simulink model "test_PCI6251_20130416_3ch"  (Simulink 7.7)
settings: Solver=ode4  StartTime=0.0  StopTime=inf  RelTol=1e-3
PreLoadFcn:
  | % Here are parameters fixed
  | % during running the real-time programs.
  | %
  | winLen=256;
  | ana_hopSize=44;
  | syn_hopSize=90;
  | 
  | nFFT=1024;
  | SampRate=44100;
  | Ts=1/SampRate;
  | 
  | % % now encoded in RealSong_control
  | %cepst_nfft=2048;    % nfft size for cepstrum.
  | %
  | %up_pitch= 8000;%
  | %low_pitch=400;%
  | %
  | %quefrency = [0:cepst_nfft]'*nFFT/(SampRate*cepst_nfft); % quefrency in [sec].
  | %quefrency_index=find((1./quefrency<up_pitch & 1./quefrency > low_pitch)); % select quefrency in 400 to 8000 Hz range.
  | 
  | 
  | %frange=[400,8000];
  | %f=SampRate*((1:nFFT)-1)/nFFT;
  | %findex=find(f>=frange(1)&f<=frange(2));
  | %entropy_frange=[1000,8000];
  | %efindex=find(f>=entropy_frange(1)&f<=entropy_frange(2));
  | 
  | 
  | mingap=1;
  | minsyl =6;
values from neighbouring files (symbols this model uses):
  amp_thresh = str2double(get(handles.edit_amp_thresh,'String'))    [RealSong_control_013.m]
  efindex = find(f>=efrange(1)&f<=efrange(2))    [RealSong_control_013.m]
  findex = find(f>=pm.frange(1)&f<=pm.frange(2))    [RealSong_control_013.m]
  mainsyl = varargin{1}    [RealSong_control_013.m]
  quefrency_index = find((1./quefrency<up_pitch & 1./quefrency > low_pitch))    [RealSong_control_013.m]
  scaling_factor = presyl.template_scaling_factor    [RealSong_control_013.m]
undefined symbols (not defined in the file or in its folder): AO1_TTL_Freq, dfilt, init_stim_vector, maindetection_startcnt, maintarget_spectrum_filter, max_presyl_cancel_counter, presyl_cntmin, svmdata
libraries: simulink x13, dspsigops x4, xpcnilib x3, dsparch4 x2, dspxfrm3 x2, IntelSMIlibR2007b x1
(part 1 of 2)
settings Model: Creator=hammer  LastModifiedBy=mooney_lab  BufferReuse=off
settings OptimizationCC: BlockReduction=off  OptimizeBlockIOStorage=off  BufferReuse=off  ExpressionFolding=off  LocalBlockOutputs=off
settings DebuggingCC: UnderspecifiedInitializationDetection=Simplified
settings HardwareCC: ProdIntDivRoundTo=Zero  ProdEndianess=LittleEndian  ProdHWDeviceType=Generic->32-bit x86 compatible
settings RTWCC: SystemTargetFile=xpctarget.tlc  TemplateMakefile=xpc_default_tmf  Description=xPC Target  RTWVerbose=off  ProcessScript=xpctarget_make_rtw_hook  RTWCompilerOptimization=On
settings xpcTargetCC: TargetFcnLib=ansi_tfl_table_tmw.mat  TargetFunctionLibrary=XPC_BLAS  FunctionExecutionProfile=off  CodeExecutionProfiling=off  ERTCodeCoverageTool=None  ParMdlRefBuildCompliant=on  CombineSignalStateStructs=off  PortableWordSizes=off  xPCTaskExecutionProfile=off  xPCRL32EventNumber=5000  xPCLoadParamSetFile=off  xPCConcurrentTasks=off  xPCEnableSFAnimation=off

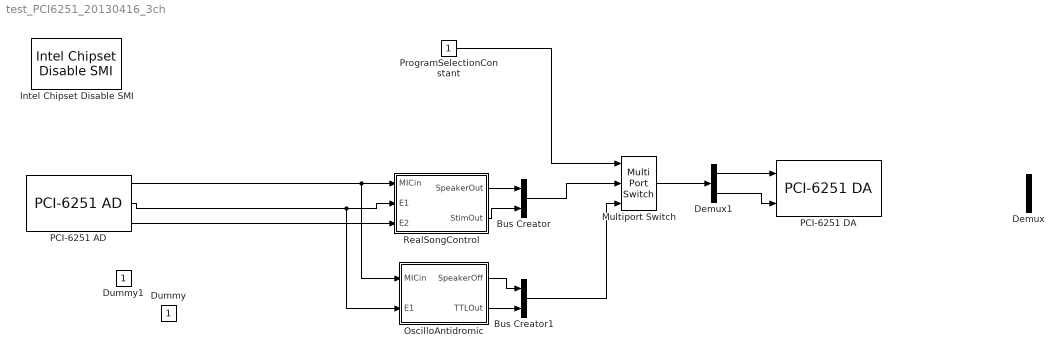
== system test_PCI6251_20130416_3ch ==
  Bus Creator : BusCreator  Inputs=2
  Bus Creator1 : BusCreator  Inputs=2
  Demux : Demux  Outputs=2
  Demux1 : Demux  Outputs=2
  Dummy : Constant  SampleTime=Ts
  Dummy1 : Constant  SampleTime=Ts
  Intel Chipset Disable SMI : IntelSMIlibR2007b/Intel Chipset Disable SMI
  Multiport Switch : MultiPortSwitch  Inputs=2  zeroidx=off
  OscilloAntidromic : Subsystem
  PCI-6251 AD : xpcnilib/A//D/M Series/PCI-6251 AD  channel=[1,2,3]  range=[10 10 10]  coupling=[0 0 0]  scantime=[4e-6, 4e-6, 4e-6]  sampletime=Ts  slot=-1
  PCI-6251 DA : xpcnilib/D//A/M Series/PCI-6251 DA  channel=[1,2]  range=[10, 10]  reset=[1, 1]  initValue=[0, 0]  sampletime=Ts  slot=-1
  ProgramSelectionConstant : Constant  SampleTime=Ts
  RealSongControl : Subsystem
  wires:
  PCI-6251 AD/1 -> RealSongControl/1(MICin), OscilloAntidromic/1(MICin)
  ProgramSelectionConstant/1 -> Multiport Switch/1
  RealSongControl/1(SpeakerOut) -> Bus Creator/1
  RealSongControl/2(StimOut) -> Bus Creator/2
  OscilloAntidromic/1(SpeakerOff) -> Bus Creator1/1
  OscilloAntidromic/2(TTLOut) -> Bus Creator1/2
  Bus Creator/1 -> Multiport Switch/2
  Bus Creator1/1 -> Multiport Switch/3
  Multiport Switch/1 -> Demux1/1
  Demux1/1 -> PCI-6251 DA/1
  Demux1/2 -> PCI-6251 DA/2
  PCI-6251 AD/2 -> RealSongControl/2(E1), OscilloAntidromic/2(E1)
  PCI-6251 AD/3 -> RealSongControl/3(E2)

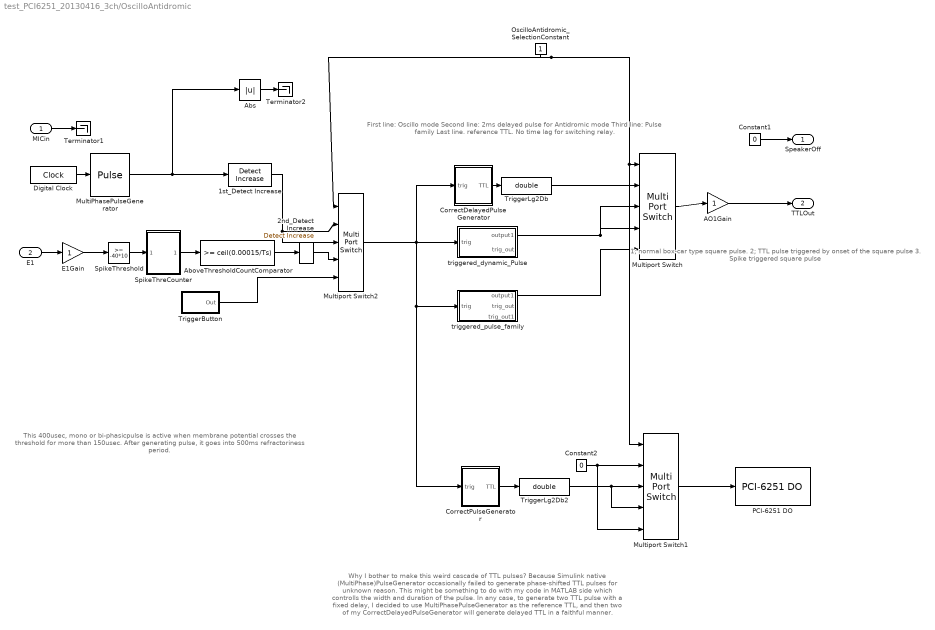
== system test_PCI6251_20130416_3ch/OscilloAntidromic ==
  note: 1; normal box-car type square pulse.
      | 2; TTL pulse triggered by onset of the square pulse
      | 3. Spike triggered square pulse
  note: First line: Oscillo mode
      | Second line: 2ms delayed pulse for Antidromic mode
      | Third line: Pulse family
      | Last line. reference TTL. No time lag for switching relay.
  note: Why I bother to make this weird cascade of TTL pulses?
      | Because Simulink native (MultiPhase)PulseGenerator occasionally failed
      | to generate phase-shifted TTL pulses for unknown reason.
      | This might be something to do with my code in MATLAB side which
      | controlls the width and duration of the pulse. In any case,
      |  to generate two TTL pulse with a fixed delay,
      | I decided to use MultiPhasePulseGenerator as the reference TTL,
      | and then two of my CorrectDelayedPulseGenerator
      | will generate delayed TTL in a faithful manner.
  note: This 400usec, mono or bi-phasicpulse is
      | active when membrane potential crosses the threshold
      | for more than 150usec. After generating pulse,
      | it goes into 500ms refractoriness period.
  MICin : Inport
  E1 : Inport  Port=2
  1st_Detect Increase : simulink/Logic and Bit Operations/Detect Increase  SystemSampleTime=-1  vinit=0.0
  2nd_Detect Increase : simulink/Logic and Bit Operations/Detect Increase  SystemSampleTime=-1  vinit=0.0
  AO1Gain : Gain
  AboveThresholdCountComparator : simulink/Logic and Bit Operations/Compare To Constant  SystemSampleTime=-1  relop=>=  const=ceil(0.00015/Ts)  LogicOutDataTypeMode=uint8
  Abs : Abs
  Constant1 : Constant  Value=0
  Constant2 : Constant  Value=0
  CorrectDelayedPulseGenerator : Subsystem  mask{maindetection_startcnt=ceil(0.002/Ts), width=ceil(0.05/Ts)}
      mask prompts: maindetection_startcnt "Delay (count)"; width "Width of TTL (count)"
  CorrectPulseGenerator : Subsystem  mask{maindetection_startcnt=0, width=ceil(0.05/Ts)}
      mask prompts: maindetection_startcnt "Delay (count)"; width "Width of TTL (count)"
  Digital Clock : DigitalClock  SampleTime=Ts
  E1Gain : Gain
  MultiPhasePulseGenerator : DiscretePulseGenerator  TimeSource=Use external signal  Period=ceil(1/AO1_TTL_Freq/Ts)  PulseWidth=ceil(0.5/AO1_TTL_Freq/Ts)  SampleTime=Ts
  Multiport Switch : MultiPortSwitch  Inputs=4  zeroidx=off
  Multiport Switch1 : MultiPortSwitch  Inputs=4  zeroidx=off
  Multiport Switch2 : MultiPortSwitch  Inputs=4  zeroidx=off
  OscilloAntidromic_SelectionConstant : Constant  SampleTime=Ts
  PCI-6251 DO : xpcnilib/Digital Output/M Series/PCI-6251 DO  channel=[1]  reset=[1]  initValue=[0]  sampletime=Ts  slot=-1
  SpikeThreCounter : Subsystem
  SpikeThreshold : simulink/Logic and Bit Operations/Compare To Constant  SystemSampleTime=-1  relop=>=  const=-40*10  LogicOutDataTypeMode=uint8
      link override Compare: Operator=<=
  Terminator1 : Terminator
  Terminator2 : Terminator
  TriggerButton : Subsystem
  TriggerLg2Db : DataTypeConversion  OutDataTypeStr=double  RndMeth=Zero
  TriggerLg2Db2 : DataTypeConversion  OutDataTypeStr=double  RndMeth=Zero
  triggered_dynamic_Pulse : Subsystem  mask{amp=1, delay=ceil(0.001/Ts), pulse_dur=ceil(0.0002/Ts), ipi=ceil(0.00021/Ts), burst_dur=ceil(0.00042/Ts), ref=ceil(0.5/Ts)}
      mask prompts: amp "Amp [V]"; delay "delay [ms]"; pulse_dur "pulse duration  [ms]"; ipi "inter_pulse_interval  [ms]"; burst_dur "total burst duration  [ms]"; ref "Ref  [ms]"
      mask init:
      | Y = make_pulse(delay,burst_dur,pulse_dur,ipi,1,44100);
      | X = 1:length(Y);
      mask Display: plot(X,Y)
  triggered_pulse_family : Subsystem  mask{delay=ceil(0.1/Ts), pulse_dur=ceil(0.1/Ts), ipi=ceil(0.4/Ts), burst_dur=ceil(1/Ts), ref=ceil(1/Ts), lowamp=-600, interval=600, highamp=600}
      mask prompts: delay "delay [ms]"; pulse_dur "pulse duration  [ms]"; ipi "inter_pulse_interval  [ms]"; burst_dur "total burst duration  [ms]"; ref "Ref  [ms]"; lowamp "Lowest current [pA]"; interval "current interval [pA]"; highamp "Highest current [pA]"
      mask init:
      | amp=[lowamp:interval:highamp]
      | if ceil(burst_dur/ipi)>length(amp)
      |     errordlg(sprintf('amp vector (%d)is shorter than required length (%d)!',...
      |         length(amp),ceil(burst_dur/ipi)));
      | end
      | 
      | Y = make_pulsefamily(delay,burst_dur,pulse_dur,ipi,amp,44100);
      | X = 1:length(Y);
      mask Display: plot(X,Y)
  SpeakerOff : Outport
  TTLOut : Outport  Port=2
  wires:
  Constant1/1 -> SpeakerOff/1
  AO1Gain/1 -> TTLOut/1
  E1/1 -> E1Gain/1
  E1Gain/1 -> SpikeThreshold/1
  MICin/1 -> Terminator1/1
  OscilloAntidromic_SelectionConstant/1 -> Multiport Switch/1, Multiport Switch1/1, Multiport Switch2/1
  Multiport Switch/1 -> AO1Gain/1
  triggered_dynamic_Pulse/1(output1) -> Multiport Switch/3, Multiport Switch/4
  Constant2/1 -> Multiport Switch1/2, Multiport Switch1/5
  Multiport Switch1/1 -> PCI-6251 DO/1
  Digital Clock/1 -> MultiPhasePulseGenerator/1
  CorrectDelayedPulseGenerator/1(TTL) -> TriggerLg2Db/1
  TriggerLg2Db/1 -> Multiport Switch/2
  TriggerLg2Db2/1 -> Multiport Switch1/4, Multiport Switch1/3
  SpikeThreshold/1 -> SpikeThreCounter/1(LogicalInput)
  SpikeThreCounter/1(count) -> AboveThresholdCountComparator/1
  Multiport Switch2/1 -> CorrectDelayedPulseGenerator/1(trig), CorrectPulseGenerator/1(trig), triggered_pulse_family/1(trig), triggered_dynamic_Pulse/1(trig)
  MultiPhasePulseGenerator/1 -> 1st_Detect Increase/1, Abs/1
  CorrectPulseGenerator/1(TTL) -> TriggerLg2Db2/1
  AboveThresholdCountComparator/1 -> 2nd_Detect Increase/1
  triggered_pulse_family/1(output1) -> Multiport Switch/5
  TriggerButton/1(Out) -> Multiport Switch2/5
  1st_Detect Increase/1 -> Multiport Switch2/3, Multiport Switch2/2
  2nd_Detect Increase/1 -> Multiport Switch2/4
  Abs/1 -> Terminator2/1

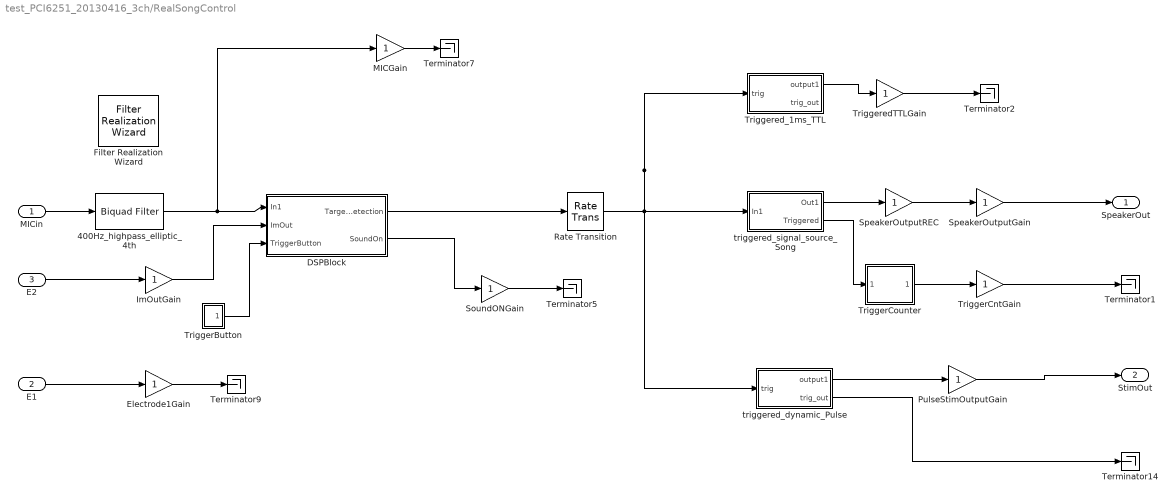
== system test_PCI6251_20130416_3ch/RealSongControl ==
  MICin : Inport
  E1 : Inport  Port=2
  E2 : Inport  Port=3
  400Hz_highpass_elliptic_4th : dsparch4/Biquad Filter  Tag=BlockMethodSubSystem  IIRFiltStruct=Direct form II  CoeffSource=Specify via dialog  BiQuadCoeffs=[1 -1.99997295416341 1 1 -1.86330921959673 0.873887398426786;1 -1.99984550773747 1 1 -1.98119934202051 0.984460391369785]  a0Flag=Warning  IC=0  ICnum=0  ICden=0  InputProcessing=Columns as channels (frame based)  denAccumFracLength=30  denProdOutputFracLength=30  secondMemoryFracLength=15  roundingMode=Floor  overflowMode=off  ScaleValues=[16.3731438660539;0.0504230422181438;1]  optimizeScaleValues=on  ScaleValueMode=Specify via input port (g)  scaleValueFracLength=14  FilterSource=Specify via dialog  dfiltObjectName=dfilt.df2tsos([1 0.3 0.4],[1 0.1 0.2])
  DSPBlock : Subsystem
  Electrode1Gain : Gain
  Filter Realization Wizard : dsparch4/Filter Realization Wizard  SystemSampleTime=-1
  ImOutGain : Gain
  MICGain : Gain
  PulseStimOutputGain : Gain
  Rate Transition : RateTransition
  SoundONGain : Gain
  SpeakerOutputGain : Gain
  SpeakerOutputREC : Gain
  Terminator{1..2,5,7,9,14} (6 alike) : Terminator
  TriggerButton : Subsystem
  TriggerCntGain : Gain
  TriggerCounter : Subsystem
  TriggeredTTLGain : Gain
  Triggered_1ms_TTL : Subsystem  mask{amp=1, delay=0.0, pulse_dur=ceil(1/1000*SampRate), ipi=ceil(1/1000*SampRate), burst_dur=ceil(1/1000*SampRate), ref=ceil(1/1000*SampRate)}
      mask prompts: amp "Amp [V]"; delay "delay [ms]"; pulse_dur "pulse duration  [ms]"; ipi "inter_pulse_interval  [ms]"; burst_dur "total burst duration  [ms]"; ref "Ref  [ms]"
      mask init:
      | Y = make_pulse(delay,burst_dur,pulse_dur,ipi,1,44100);
      | X = 1:length(Y);
      mask Display: plot(X,Y)
  triggered_dynamic_Pulse : Subsystem  mask{amp=1, delay=0, pulse_dur=ceil(0.4/1000*SampRate), ipi=ceil(1/1000*SampRate), burst_dur=ceil(4/1000*SampRate), ref=ceil(100/1000*SampRate)}
      mask prompts: amp "Amp [V]"; delay "delay [ms]"; pulse_dur "pulse duration  [ms]"; ipi "inter_pulse_interval  [ms]"; burst_dur "total burst duration  [ms]"; ref "Ref  [ms]"
      mask init:
      | Y = make_pulse(delay,burst_dur,pulse_dur,ipi,1,44100);
      | X = 1:length(Y);
      mask Display: plot(X,Y)
  triggered_signal_source_Song : Subsystem  mask{OutValues=init_stim_vector, ref=length(init_stim_vector), on_off=1}
      mask prompts: OutValues "Output Values"; on_off "ON/Off"
      mask init:
      | dim = size(OutValues);
      | if length(dim) > 2 || min(dim) ~= 1
      |   [X, Y] =  generateQuestionMarkIconData;
      | error('Parameter ''output values'' must be a vector or a scalar');
      |   else
      |   nn = length(OutValues);
      |   xx = (0:nn);
      |   yy = double([reshape(OutValues,1,nn) OutValues(end)]);
      |  X = fixpt_look1_mask_data(xx,yy,1,4);
      |  Y = fixpt_look1_mask_data(xx,yy,0,4);
      |  end
      mask Display: plot(X,Y)
  SpeakerOut : Outport
  StimOut : Outport  Port=2
  wires:
  triggered_signal_source_Song/1(Out1) -> SpeakerOutputREC/1
  triggered_signal_source_Song/2(Triggered) -> TriggerCounter/1(LogicalInput)
  TriggerCounter/1(count) -> TriggerCntGain/1
  MICGain/1 -> Terminator7/1
  SpeakerOutputGain/1 -> SpeakerOut/1
  E1/1 -> Electrode1Gain/1
  Electrode1Gain/1 -> Terminator9/1
  PulseStimOutputGain/1 -> StimOut/1
  triggered_dynamic_Pulse/1(output1) -> PulseStimOutputGain/1
  triggered_dynamic_Pulse/2(trig_out) -> Terminator14/1
  SoundONGain/1 -> Terminator5/1
  TriggerCntGain/1 -> Terminator1/1
  TriggeredTTLGain/1 -> Terminator2/1
  Triggered_1ms_TTL/1(output1) -> TriggeredTTLGain/1
  DSPBlock/2(SoundOn) -> SoundONGain/1
  400Hz_highpass_elliptic_4th/1 -> DSPBlock/1(In1), MICGain/1
  MICin/1 -> 400Hz_highpass_elliptic_4th/1
  SpeakerOutputREC/1 -> SpeakerOutputGain/1
  Rate Transition/1 -> triggered_dynamic_Pulse/1(trig), triggered_signal_source_Song/1(In1), Triggered_1ms_TTL/1(trig)
  TriggerButton/1(Out1) -> DSPBlock/3(TriggerButton)
  E2/1 -> ImOutGain/1
  ImOutGain/1 -> DSPBlock/2(ImOut)
  DSPBlock/1(TargetSyllableDetection) -> Rate Transition/1

== system test_PCI6251_20130416_3ch/OscilloAntidromic/CorrectDelayedPulseGenerator ==
  trig : Inport
  Delayed TTL generator : Stateflow chart  TreatAsAtomicUnit=on
  delay : Constant  Value=maindetection_startcnt  VectorParams1D=off
  width : Constant  Value=width  VectorParams1D=off
  TTL : Outport
  wires:
  delay/1 -> Delayed TTL generator/2(delays)
  width/1 -> Delayed TTL generator/3(width)
  trig/1 -> Delayed TTL generator/1(trig)
  Delayed TTL generator/1(out) -> TTL/1

== system test_PCI6251_20130416_3ch/OscilloAntidromic/CorrectPulseGenerator ==
  trig : Inport
  Delayed TTL generator : Stateflow chart  TreatAsAtomicUnit=on
  delay : Constant  Value=maindetection_startcnt  VectorParams1D=off
  width : Constant  Value=width  VectorParams1D=off
  TTL : Outport
  wires:
  delay/1 -> Delayed TTL generator/2(delays)
  width/1 -> Delayed TTL generator/3(width)
  trig/1 -> Delayed TTL generator/1(trig)
  Delayed TTL generator/1(out) -> TTL/1

== system test_PCI6251_20130416_3ch/OscilloAntidromic/SpikeThreCounter ==
  LogicalInput : Inport
  Counter : Subsystem  TreatAsAtomicUnit=on
  Data Type Conversion1 : DataTypeConversion  OutDataTypeStr=double  RndMeth=Zero
  count : Outport
  wires:
  Data Type Conversion1/1 -> Counter/1(In1)
  LogicalInput/1 -> Data Type Conversion1/1, Counter/Enable
  Counter/1(Out1) -> count/1

== system test_PCI6251_20130416_3ch/OscilloAntidromic/TriggerButton ==
  Detect Change : simulink/Logic and Bit Operations/Detect Change  SystemSampleTime=-1  vinit=1.0
  TrigVal : Constant  Value=1.0  OutDataTypeStr=int8
  TriggerLg2Db : DataTypeConversion  OutDataTypeStr=double  RndMeth=Zero
  Out : Outport
  wires:
  Detect Change/1 -> TriggerLg2Db/1
  TrigVal/1 -> Detect Change/1
  TriggerLg2Db/1 -> Out/1

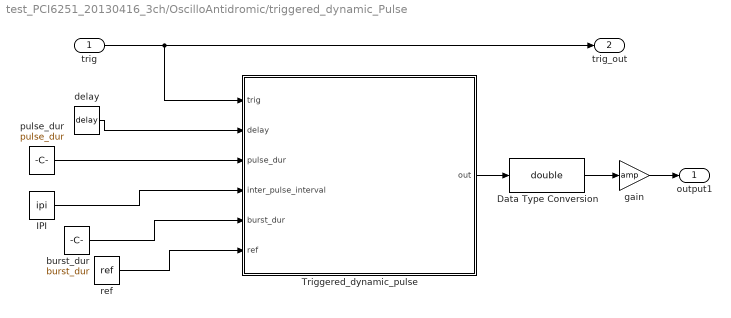
== system test_PCI6251_20130416_3ch/OscilloAntidromic/triggered_dynamic_Pulse ==
  trig : Inport
  Data Type Conversion : DataTypeConversion  OutDataTypeStr=double
  IPI : Constant  Value=ipi
  Triggered_dynamic_pulse : Stateflow chart  TreatAsAtomicUnit=on
  burst_dur : Constant  Value=burst_dur
  delay : Constant  Value=delay
  gain : Gain  Gain=amp
  pulse_dur : Constant  Value=pulse_dur
  ref : Constant  Value=ref
  output1 : Outport
  trig_out : Outport  Port=2
  wires:
  delay/1 -> Triggered_dynamic_pulse/2(delay)
  pulse_dur/1 -> Triggered_dynamic_pulse/3(pulse_dur)
  IPI/1 -> Triggered_dynamic_pulse/4(inter_pulse_interval)
  burst_dur/1 -> Triggered_dynamic_pulse/5(burst_dur)
  ref/1 -> Triggered_dynamic_pulse/6(ref)
  trig/1 -> Triggered_dynamic_pulse/1(trig), trig_out/1
  Triggered_dynamic_pulse/1(out) -> Data Type Conversion/1
  Data Type Conversion/1 -> gain/1
  gain/1 -> output1/1

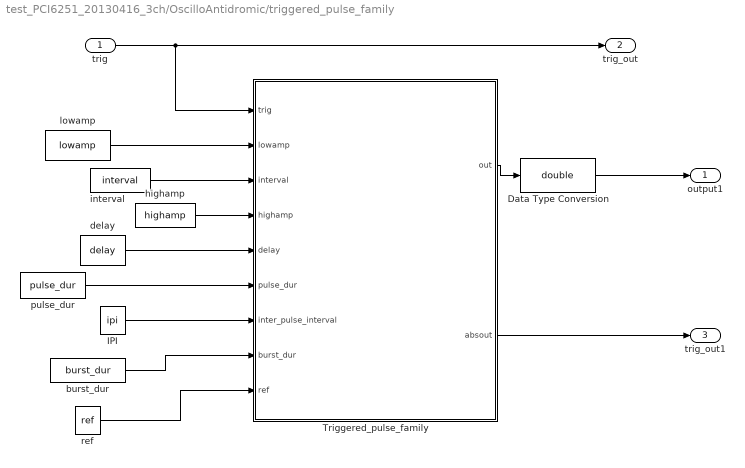
== system test_PCI6251_20130416_3ch/OscilloAntidromic/triggered_pulse_family ==
  trig : Inport
  Data Type Conversion : DataTypeConversion  OutDataTypeStr=double
  IPI : Constant  Value=ipi
  Triggered_pulse_family : Stateflow chart  TreatAsAtomicUnit=on
  burst_dur : Constant  Value=burst_dur
  delay : Constant  Value=delay
  highamp : Constant  Value=highamp
  interval : Constant  Value=interval
  lowamp : Constant  Value=lowamp
  pulse_dur : Constant  Value=pulse_dur
  ref : Constant  Value=ref
  output1 : Outport
  trig_out : Outport  Port=2
  trig_out1 : Outport  Port=3
  wires:
  delay/1 -> Triggered_pulse_family/5(delay)
  pulse_dur/1 -> Triggered_pulse_family/6(pulse_dur)
  IPI/1 -> Triggered_pulse_family/7(inter_pulse_interval)
  burst_dur/1 -> Triggered_pulse_family/8(burst_dur)
  ref/1 -> Triggered_pulse_family/9(ref)
  trig/1 -> Triggered_pulse_family/1(trig), trig_out/1
  Triggered_pulse_family/1(out) -> Data Type Conversion/1
  Data Type Conversion/1 -> output1/1
  lowamp/1 -> Triggered_pulse_family/2(lowamp)
  interval/1 -> Triggered_pulse_family/3(interval)
  highamp/1 -> Triggered_pulse_family/4(highamp)
  Triggered_pulse_family/2(absout) -> trig_out1/1

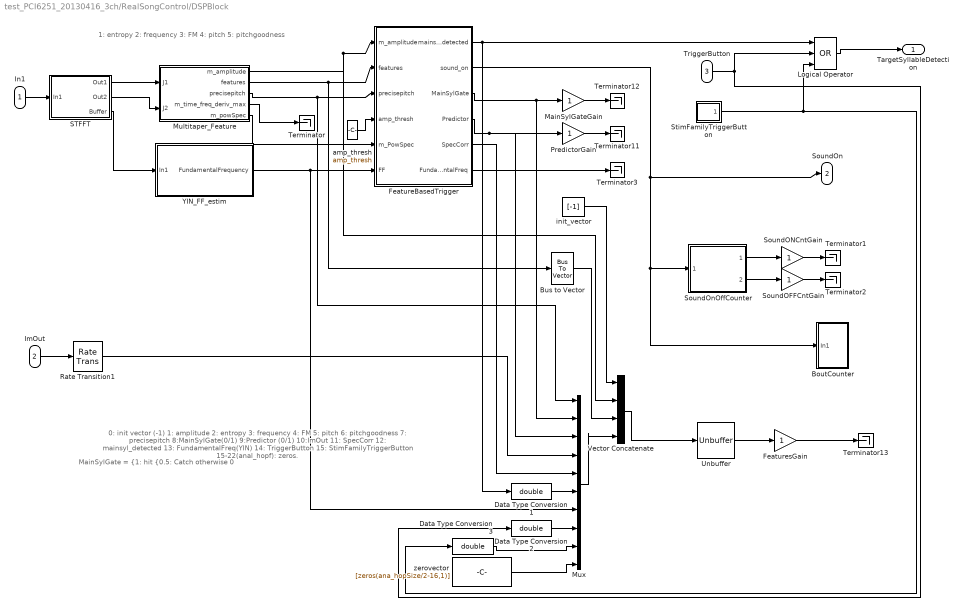
== system test_PCI6251_20130416_3ch/RealSongControl/DSPBlock ==
  note: 1: entropy
      | 2: frequency
      | 3: FM
      | 4: pitch
      | 5: pitchgoodness
  note: 0: init vector (-1)
      | 1: amplitude
      | 2: entropy
      | 3: frequency
      | 4: FM
      | 5: pitch
      | 6: pitchgoodness
      | 7: precisepitch
      | 8:MainSylGate(0/1)
      | 9:Predictor (0/1)
      | 10:ImOut
      | 11: SpecCorr
      | 12: mainsyl_detected
      | 13: FundamentalFreq(YIN)
      | 14: TriggerButton
      | 15: StimFamilyTriggerButton
      | 15-22(anal_hopf): zeros.
  note: MainSylGate =
      |  {1:  hit
      |           {0.5: Catch
      | otherwise 0
  In1 : Inport
  ImOut : Inport  Port=2
  TriggerButton : Inport  Port=3
  BoutCounter : Subsystem
  Bus to Vector : BusToVector
  Data Type Conversion1 : DataTypeConversion  OutDataTypeStr=double  RndMeth=Zero
  Data Type Conversion2 : DataTypeConversion  OutDataTypeStr=double  RndMeth=Zero
  Data Type Conversion3 : DataTypeConversion  OutDataTypeStr=double  RndMeth=Zero
  FeatureBasedTrigger : Subsystem
  FeaturesGain : Gain
  Logical Operator : Logic  Operator=OR  Inputs=3  AllPortsSameDT=off  OutDataTypeStr=boolean
  MainSylGateGain : Gain
  Multitaper_Feature : Subsystem  mask{Ts=Ts, findex=findex, efindex=efindex, quefrency_index=quefrency_index}
      mask prompts: Ts "Sample Time"; findex "Frequency index"; efindex "Frequency index for Entropy"; quefrency_index "Quefrency index"
  Mux : Mux  Inputs=10
  PredictorGain : Gain
  Rate Transition1 : RateTransition
  STFFT : Subsystem
      mask Display: disp('Overlap\nST-FFT')
  SoundOFFCntGain : Gain
  SoundONCntGain : Gain
  SoundOnOffCounter : Subsystem
  StimFamilyTriggerButton : Subsystem
  Terminator{,1..3,11..13} (7 alike) : Terminator
  Unbuffer : Unbuffer  SampleBasedProcessing=Same as frame based
  Vector Concatenate : Concatenate  NumInputs=4  Mode=Vector
  YIN_FF_estim : Subsystem  mask{SampRate=SampRate, WinT=4, lagT=1.5, lag_index=0, W_index=0}
      mask prompts: SampRate "Sampling Rate"; WinT "Window size [ms]"; lagT "Search period [ms]"
      mask init:
      | nx = 256;
      | 
      | nW=ceil(WinT/1000*SampRate);
      | nlag=ceil(lagT/1000*SampRate);
      | 
      | W_index=0:(nW-1);
      | W_index = nx-W_index;
      | 
      | lag_index = nW+[0:(nlag-1)];
      | lag_index = nx-lag_index;
  amp_thresh : Constant  Value=amp_thresh
  init_vector : Constant  Value=[-1]
  zerovector : Constant  Value=[zeros(ana_hopSize/2-16,1)]
  TargetSyllableDetection : Outport
  SoundOn : Outport  Port=2
  wires:
  STFFT/1(Out1) -> Multitaper_Feature/1(J1)
  STFFT/2(Out2) -> Multitaper_Feature/2(J2)
  Multitaper_Feature/2(features) -> FeatureBasedTrigger/2(features), Bus to Vector/1
  Multitaper_Feature/3(precisepitch) -> FeatureBasedTrigger/3(precisepitch), Mux/1
  Multitaper_Feature/1(m_amplitude) -> FeatureBasedTrigger/1(m_amplitude), Vector Concatenate/2
  FeatureBasedTrigger/2(sound_on) -> SoundOn/1, SoundOnOffCounter/1(SoundOn), BoutCounter/1(In1)
  Multitaper_Feature/4(m_time_freq_deriv_max) -> Terminator/1
  SoundOnOffCounter/1(SoundONCnt) -> SoundONCntGain/1
  SoundOnOffCounter/2(SoundOFFCnt) -> SoundOFFCntGain/1
  SoundONCntGain/1 -> Terminator1/1
  SoundOFFCntGain/1 -> Terminator2/1
  FeatureBasedTrigger/3(MainSylGate) -> MainSylGateGain/1, Mux/2
  FeatureBasedTrigger/4(Predictor) -> PredictorGain/1, Mux/3
  amp_thresh/1 -> FeatureBasedTrigger/4(amp_thresh)
  FeaturesGain/1 -> Terminator13/1
  In1/1 -> STFFT/1(In1)
  FeatureBasedTrigger/1(mainsyl_detected) -> Data Type Conversion1/1, Logical Operator/1
  Vector Concatenate/1 -> Unbuffer/1
  Unbuffer/1 -> FeaturesGain/1
  Mux/1 -> Vector Concatenate/4
  MainSylGateGain/1 -> Terminator12/1
  PredictorGain/1 -> Terminator11/1
  Bus to Vector/1 -> Vector Concatenate/3
  init_vector/1 -> Vector Concatenate/1
  Multitaper_Feature/5(m_powSpec) -> FeatureBasedTrigger/5(m_PowSpec)
  ImOut/1 -> Rate Transition1/1
  zerovector/1 -> Mux/10
  Rate Transition1/1 -> Mux/4
  FeatureBasedTrigger/5(SpecCorr) -> Mux/5
  Data Type Conversion1/1 -> Mux/6
  YIN_FF_estim/1(FundamentalFrequency) -> FeatureBasedTrigger/6(FF), Mux/7
  FeatureBasedTrigger/6(FundamentalFreq) -> Terminator3/1
  STFFT/3(Buffer) -> YIN_FF_estim/1(In1)
  Logical Operator/1 -> TargetSyllableDetection/1
  TriggerButton/1 -> Logical Operator/2, Data Type Conversion2/1
  Data Type Conversion2/1 -> Mux/8
  StimFamilyTriggerButton/1(Out1) -> Logical Operator/3, Data Type Conversion3/1
  Data Type Conversion3/1 -> Mux/9

== system test_PCI6251_20130416_3ch/RealSongControl/TriggerButton ==
  Detect Change : simulink/Logic and Bit Operations/Detect Change  SystemSampleTime=-1  vinit=1.0
  TrigVal : Constant  Value=1.0  OutDataTypeStr=int8
  Out1 : Outport
  wires:
  Detect Change/1 -> Out1/1
  TrigVal/1 -> Detect Change/1

== system test_PCI6251_20130416_3ch/RealSongControl/TriggerCounter ==
  LogicalInput : Inport
  Counter : Subsystem  TreatAsAtomicUnit=on
  Data Type Conversion1 : DataTypeConversion  OutDataTypeStr=uint8  RndMeth=Zero
  count : Outport
  wires:
  Data Type Conversion1/1 -> Counter/1(In1)
  LogicalInput/1 -> Data Type Conversion1/1, Counter/Enable
  Counter/1(Out1) -> count/1

== system test_PCI6251_20130416_3ch/RealSongControl/Triggered_1ms_TTL ==
  trig : Inport
  Data Type Conversion : DataTypeConversion  OutDataTypeStr=double
  IPI : Constant  Value=ipi
  Triggered_dynamic_pulse : Stateflow chart  TreatAsAtomicUnit=on
  burst_dur : Constant  Value=burst_dur
  delay : Constant  Value=delay
  gain : Gain  Gain=amp
  pulse_dur : Constant  Value=pulse_dur
  ref : Constant  Value=ref
  output1 : Outport
  trig_out : Outport  Port=2
  wires:
  delay/1 -> Triggered_dynamic_pulse/2(delay)
  pulse_dur/1 -> Triggered_dynamic_pulse/3(pulse_dur)
  IPI/1 -> Triggered_dynamic_pulse/4(inter_pulse_interval)
  burst_dur/1 -> Triggered_dynamic_pulse/5(burst_dur)
  ref/1 -> Triggered_dynamic_pulse/6(ref)
  trig/1 -> Triggered_dynamic_pulse/1(trig), trig_out/1
  Triggered_dynamic_pulse/1(out) -> Data Type Conversion/1
  Data Type Conversion/1 -> gain/1
  gain/1 -> output1/1

== system test_PCI6251_20130416_3ch/RealSongControl/triggered_dynamic_Pulse ==
  trig : Inport
  Data Type Conversion : DataTypeConversion  OutDataTypeStr=double
  IPI : Constant  Value=ipi
  Triggered_dynamic_pulse : Stateflow chart  TreatAsAtomicUnit=on
  burst_dur : Constant  Value=burst_dur
  delay : Constant  Value=delay
  gain : Gain  Gain=amp
  pulse_dur : Constant  Value=pulse_dur
  ref : Constant  Value=ref
  output1 : Outport
  trig_out : Outport  Port=2
  wires:
  delay/1 -> Triggered_dynamic_pulse/2(delay)
  pulse_dur/1 -> Triggered_dynamic_pulse/3(pulse_dur)
  IPI/1 -> Triggered_dynamic_pulse/4(inter_pulse_interval)
  burst_dur/1 -> Triggered_dynamic_pulse/5(burst_dur)
  ref/1 -> Triggered_dynamic_pulse/6(ref)
  trig/1 -> Triggered_dynamic_pulse/1(trig), trig_out/1
  Triggered_dynamic_pulse/1(out) -> Data Type Conversion/1
  Data Type Conversion/1 -> gain/1
  gain/1 -> output1/1

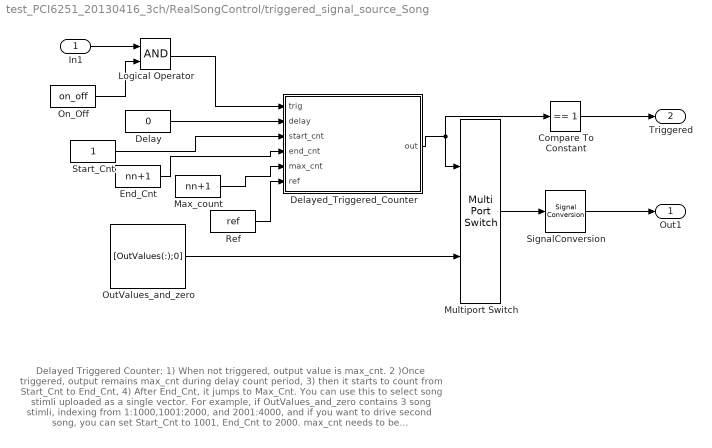
== system test_PCI6251_20130416_3ch/RealSongControl/triggered_signal_source_Song ==
  note: Delayed Triggered Counter:
      | 1) When not triggered, output value is max_cnt.
      | 2 )Once triggered, output remains max_cnt
      | during delay count period,
      | 3) then it starts to count from
      | Start_Cnt to End_Cnt,
      | 4) After End_Cnt, it jumps to Max_Cnt.
      |
      | You can use this to select song stimli uploaded as
      | a single vector. For example, if OutValues_and_zero contains
      | 3 song stimli, indexing from 1:1000,1001:2000, and 2001:4000,
      | and if you want to drive second song, you can set Start_Cnt to 1001, End_Cnt to 2000.
      | max_cnt needs to be length(OutValues_and_zero)+1 to make sure
      | the analog output goes back to zero.
  In1 : Inport
  Compare To Constant : simulink/Logic and Bit Operations/Compare To Constant  SystemSampleTime=-1  relop===  const=1  LogicOutDataTypeMode=uint8
  Delay : Constant  Value=0
  Delayed_Triggered_Counter : Stateflow chart  TreatAsAtomicUnit=on
  End_Cnt : Constant  Value=nn+1
  Logical Operator : Logic  AllPortsSameDT=off  OutDataTypeStr=boolean
  Max_count : Constant  Value=nn+1
  Multiport Switch : MultiPortSwitch  Inputs=1  zeroidx=off
  On_Off : Constant  Value=on_off
  OutValues_and_zero : Constant  Value=[OutValues(:);0]
  Ref : Constant  Value=ref
  SignalConversion : SignalConversion  ConversionOutput=Contiguous copy
  Start_Cnt : Constant
  Out1 : Outport
  Triggered : Outport  Port=2
  wires:
  Max_count/1 -> Delayed_Triggered_Counter/5(max_cnt)
  Delayed_Triggered_Counter/1(out) -> Multiport Switch/1, Compare To Constant/1
  OutValues_and_zero/1 -> Multiport Switch/2
  Multiport Switch/1 -> SignalConversion/1
  SignalConversion/1 -> Out1/1
  Ref/1 -> Delayed_Triggered_Counter/6(ref)
  Compare To Constant/1 -> Triggered/1
  In1/1 -> Logical Operator/1
  On_Off/1 -> Logical Operator/2
  Logical Operator/1 -> Delayed_Triggered_Counter/1(trig)
  Delay/1 -> Delayed_Triggered_Counter/2(delay)
  Start_Cnt/1 -> Delayed_Triggered_Counter/3(start_cnt)
  End_Cnt/1 -> Delayed_Triggered_Counter/4(end_cnt)

== system test_PCI6251_20130416_3ch/OscilloAntidromic/SpikeThreCounter/Counter ==
  In1 : Inport
  Enable : EnablePort  StatesWhenEnabling=reset
  Memory1 : Memory  InheritSampleTime=on
  Sum1 : Sum  Inputs=|++  SaturateOnIntegerOverflow=on
  Out1 : Outport  OutputWhenDisabled=reset  InitialOutput=0
  wires:
  In1/1 -> Sum1/1
  Sum1/1 -> Out1/1, Memory1/1
  Memory1/1 -> Sum1/2

== system test_PCI6251_20130416_3ch/RealSongControl/DSPBlock/BoutCounter ==
  In1 : Inport
  BoutDurCounter : Subsystem  mask{mingap=ceil(0.2*SampRate/ana_hopSize), minsyl=ceil(0.03*SampRate/ana_hopSize)}
      mask prompts: mingap "Gap shorter than this is neglected"; minsyl "On state must be longer than this"
  BoutONGAINSEC : Gain  Gain=ana_hopSize*Ts
  BoutONGain : Gain
  BoutThresh : Constant  Value=0.5
  CorrectDelayedPulseGenerator forRecordingEnableSignal : Subsystem  mask{maindetection_startcnt=1, width=ceil(SampRate/ana_hopSize)}
      mask prompts: maindetection_startcnt "Delay (count)"; width "Width of TTL (count)"
  IsBoutLongEnough : RelationalOperator  Operator=>  OutDataTypeStr=boolean
  MinBoutDur : Constant  Value=0.8
  RECGain : Gain
  Terminator4 : Terminator
  Terminator8 : Terminator
  wires:
  BoutDurCounter/1(SignalOn) -> BoutONGain/1
  BoutDurCounter/2(SignalOnCnt) -> BoutONGAINSEC/1
  BoutThresh/1 -> BoutDurCounter/2(threshold)
  BoutONGAINSEC/1 -> IsBoutLongEnough/1
  IsBoutLongEnough/1 -> CorrectDelayedPulseGenerator forRecordingEnableSignal/1(trig)
  MinBoutDur/1 -> IsBoutLongEnough/2
  CorrectDelayedPulseGenerator forRecordingEnableSignal/1(TTL) -> RECGain/1
  BoutONGain/1 -> Terminator4/1
  RECGain/1 -> Terminator8/1
  In1/1 -> BoutDurCounter/1(Input)

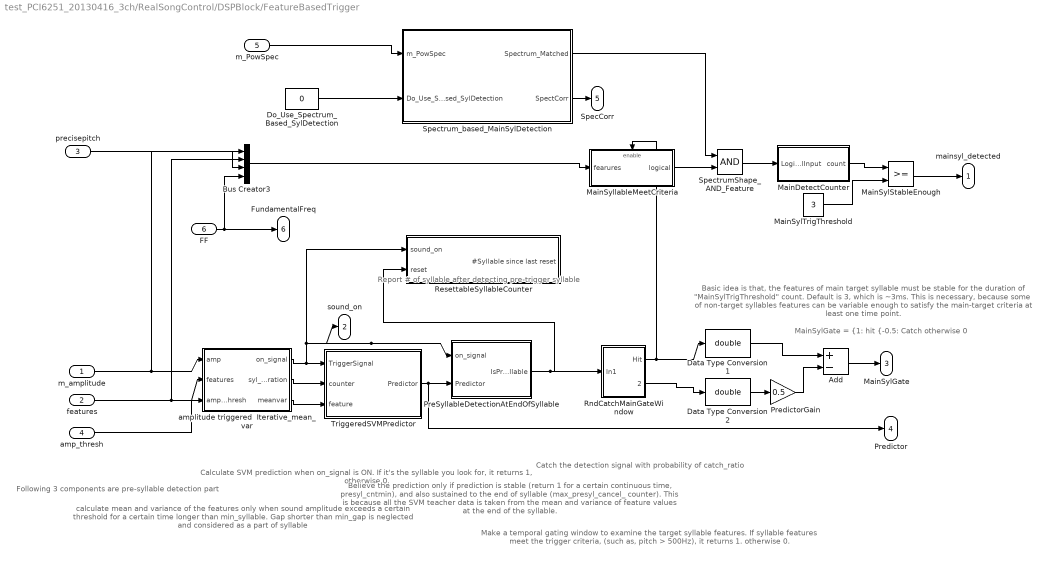
== system test_PCI6251_20130416_3ch/RealSongControl/DSPBlock/FeatureBasedTrigger ==
  note: Calculate SVM prediction
      | when on_signal is ON.
      | If it's the syllable you look for,
      | it returns 1,
      | otherwise 0.
  note: calculate mean and variance
      | of the features only when sound amplitude
      | exceeds a certain threshold for a certain time
      | longer than min_syllable. Gap shorter than
      | min_gap is neglected and considered
      | as a part of syllable
  note: Believe the prediction
      | only if prediction is stable
      | (return 1 for a certain continuous
      |  time, presyl_cntmin),
      | and also sustained to the end of
      | syllable (max_presyl_cancel_
      | counter). This is because all the
      | SVM teacher data is taken from
      | the mean and variance of feature
      | values at the end of the syllable.
  note: Make a temporal gating window
      | to examine the target syllable
      | features. If syllable features
      | meet the trigger criteria,
      | (such as, pitch > 500Hz),
      | it returns 1.
      | otherwise 0.
  note: Following 3 components are
      | pre-syllable detection part
  note: Report # of syllable after detecting
      | pre-trigger syllable
  note: Catch the detection
      | signal with probability
      | of catch_ratio
  note: Basic idea is that,
      | the features of main target syllable
      | must be stable for the duration of
      | "MainSylTrigThreshold" count.
      | Default is 3, which is ~3ms.
      |
      | This is necessary, because some of
      | non-target syllables features can be
      | variable enough to satisfy the
      | main-target criteria at least one time point.
  note: MainSylGate =
      |  {1:  hit
      |           {-0.5: Catch
      | otherwise 0
  m_amplitude : Inport
  features : Inport  Port=2
  precisepitch : Inport  Port=3
  amp_thresh : Inport  Port=4
  m_PowSpec : Inport  Port=5
  FF : Inport  Port=6
  Add : Sum  Inputs=+-
  Bus Creator3 : BusCreator
  Data Type Conversion1 : DataTypeConversion  OutDataTypeStr=double  RndMeth=Zero
  Data Type Conversion2 : DataTypeConversion  OutDataTypeStr=double  RndMeth=Zero
  Do_Use_Spectrum_Based_SylDetection : Constant  Value=0
  MainDetectCounter : Subsystem
  MainSylStableEnough : RelationalOperator  OutDataTypeStr=boolean
  MainSylTrigThreshold : Constant  Value=3
  MainSyllableMeetCriteria : Subsystem  TreatAsAtomicUnit=on  mask{criteria=mainsyl.criteria}
      mask prompts: criteria "Main Syllable Trigger Criteria"
  PreSyllableDetectionAtEndOfSyllable : Subsystem  mask{presyl_cntmin=presyl_cntmin, max_presyl_cancel_counter=max_presyl_cancel_counter}
      mask prompts: presyl_cntmin "Minimum PreSyllable Prediction Count"; max_presyl_cancel_counter "Max PreSyllable Cancel Counter"
  PredictorGain : Gain  Gain=0.5
  ResettableSyllableCounter : Subsystem
  RndCatchMainGateWindow : Subsystem
  SpectrumShape_ AND_Feature : Logic  AllPortsSameDT=off  OutDataTypeStr=boolean
  Spectrum_based_MainSylDetection : Subsystem  mask{maintarget_spectrum_filter=maintarget_spectrum_filter, Spectrum_Filter_Threshold=1}
      mask prompts: maintarget_spectrum_filter "Spectrum Filter (length is same as findex, needs to be normalized with STD)"; Spectrum_Filter_Threshold "Spectrum Filter Threshold"
      mask init:
      | % % 
      | % if length(maintarget_spectrum_filter)~= length(findex)
      | % error('Size of ''maintarget_spectrum_filter'' must be same as findex');
      | % end
      | 
      | % normalize to make the correlation coefficient 
      | % bounded within -1 to 1.
      | %  
      | % if std(maintarget_spectrum_filter)~= 1
      | % maintarget_spectrum_filter = maintarget_spectrum_filter/std(maintarget_spectrum_filter);
      | % end
      mask Display: plot(findex,maintarget_spectrum_filter);
  TriggeredSVMPredictor : Subsystem  mask{svmdata=svmdata, scaling_factor=scaling_factor}
      mask prompts: svmdata "SVM Data"; scaling_factor "Scaling factor"
  amplitude triggered  Iterative_mean_var : Subsystem  mask{minsyl=minsyl, mingap=mingap}
      mask prompts: minsyl "Minimum syllable count"; mingap "Minimum gap count"
      mask help:
      | If amp > amp_thresh,  start counter and reset gap counter.
      | Else, start gap counter and reset counter.
      |
      | If counter > minimum syllable count, and
      | If gap counter < minimum gap count,
      |
      | It is considered as above threshold, and starts to calculate
      | mean and variance of the features.
  mainsyl_detected : Outport
  sound_on : Outport  Port=2
  MainSylGate : Outport  Port=3
  Predictor : Outport  Port=4
  SpecCorr : Outport  Port=5
  FundamentalFreq : Outport  Port=6
  wires:
  Bus Creator3/1 -> MainSyllableMeetCriteria/1(fearures)
  PreSyllableDetectionAtEndOfSyllable/1(IsPreSyllable) -> ResettableSyllableCounter/2(reset), RndCatchMainGateWindow/1(In1)
  TriggeredSVMPredictor/1(Predictor) -> PreSyllableDetectionAtEndOfSyllable/2(Predictor), Predictor/1
  amplitude triggered  Iterative_mean_var/3(meanvar) -> TriggeredSVMPredictor/3(feature)
  amplitude triggered  Iterative_mean_var/2(syl_duration) -> TriggeredSVMPredictor/2(counter)
  amplitude triggered  Iterative_mean_var/1(on_signal) -> PreSyllableDetectionAtEndOfSyllable/1(on_signal), sound_on/1, ResettableSyllableCounter/1(sound_on), TriggeredSVMPredictor/1(TriggerSignal)
  features/1 -> Bus Creator3/2, amplitude triggered  Iterative_mean_var/2(features)
  precisepitch/1 -> Bus Creator3/3
  RndCatchMainGateWindow/1(Hit) -> MainSyllableMeetCriteria/Enable, Data Type Conversion1/1
  m_amplitude/1 -> Bus Creator3/1, amplitude triggered  Iterative_mean_var/1(amp)
  amp_thresh/1 -> amplitude triggered  Iterative_mean_var/3(amp_thresh)
  MainDetectCounter/1(count) -> MainSylStableEnough/1
  MainSylTrigThreshold/1 -> MainSylStableEnough/2
  MainSylStableEnough/1 -> mainsyl_detected/1
  RndCatchMainGateWindow/2(Catch) -> Data Type Conversion2/1
  Data Type Conversion2/1 -> PredictorGain/1
  Data Type Conversion1/1 -> Add/1
  PredictorGain/1 -> Add/2
  Add/1 -> MainSylGate/1
  m_PowSpec/1 -> Spectrum_based_MainSylDetection/1(m_PowSpec)
  Spectrum_based_MainSylDetection/1(Spectrum_Matched) -> SpectrumShape_ AND_Feature/1
  SpectrumShape_ AND_Feature/1 -> MainDetectCounter/1(LogicalInput)
  MainSyllableMeetCriteria/1(logical) -> SpectrumShape_ AND_Feature/2
  Do_Use_Spectrum_Based_SylDetection/1 -> Spectrum_based_MainSylDetection/2(Do_Use_Spectrum_Based_SylDetection)
  Spectrum_based_MainSylDetection/2(SpectCorr) -> SpecCorr/1
  FF/1 -> FundamentalFreq/1, Bus Creator3/4

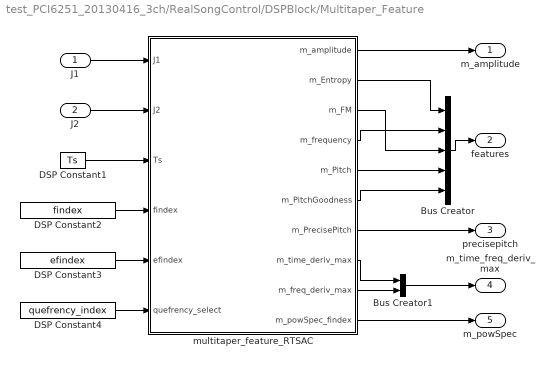
== system test_PCI6251_20130416_3ch/RealSongControl/DSPBlock/Multitaper_Feature ==
  J1 : Inport
  J2 : Inport  Port=2
  Bus Creator : BusCreator  Inputs=5
  Bus Creator1 : BusCreator  Inputs=2
  DSP Constant1 : Constant  Value=Ts  VectorParams1D=off
  DSP Constant2 : Constant  Value=findex  VectorParams1D=off
  DSP Constant3 : Constant  Value=efindex  VectorParams1D=off
  DSP Constant4 : Constant  Value=quefrency_index  VectorParams1D=off
  multitaper_feature_RTSAC : Stateflow chart  TreatAsAtomicUnit=on
  m_amplitude : Outport
  features : Outport  Port=2
  precisepitch : Outport  Port=3
  m_time_freq_deriv_max : Outport  Port=4
  m_powSpec : Outport  Port=5
  wires:
  DSP Constant1/1 -> multitaper_feature_RTSAC/3(Ts)
  DSP Constant2/1 -> multitaper_feature_RTSAC/4(findex)
  multitaper_feature_RTSAC/2(m_Entropy) -> Bus Creator/1
  DSP Constant3/1 -> multitaper_feature_RTSAC/5(efindex)
  multitaper_feature_RTSAC/1(m_amplitude) -> m_amplitude/1
  J1/1 -> multitaper_feature_RTSAC/1(J1)
  J2/1 -> multitaper_feature_RTSAC/2(J2)
  Bus Creator/1 -> features/1
  multitaper_feature_RTSAC/7(m_PrecisePitch) -> precisepitch/1
  multitaper_feature_RTSAC/8(m_time_deriv_max) -> Bus Creator1/1
  multitaper_feature_RTSAC/9(m_freq_deriv_max) -> Bus Creator1/2
  Bus Creator1/1 -> m_time_freq_deriv_max/1
  multitaper_feature_RTSAC/5(m_Pitch) -> Bus Creator/4
  multitaper_feature_RTSAC/6(m_PitchGoodness) -> Bus Creator/5
  multitaper_feature_RTSAC/4(m_frequency) -> Bus Creator/2
  multitaper_feature_RTSAC/3(m_FM) -> Bus Creator/3
  DSP Constant4/1 -> multitaper_feature_RTSAC/6(quefrency_select)
  multitaper_feature_RTSAC/10(m_powSpec_findex) -> m_powSpec/1

== system test_PCI6251_20130416_3ch/RealSongControl/DSPBlock/STFFT ==
  In1 : Inport
  Analysis Window : dspsigops/Window Function  winmode=Apply window to input  wintype=User defined  sampmode=Continuous  samptime=1  N=64  Rs=50  beta=10  winsamp=Periodic  UserWindow=dpss_return  OptParams=on  UserParams={1}  RowConvenienceOn=on  dataType=double  isSigned=on  wordLen=16  udDataType=sfix(16)  fracBitsMode=Best precision  numFracBits=15  roundingMode=Floor  overflowMode=off  numSidelobes=4  sidelobeLevel=-30
  Analysis Window1 : dspsigops/Window Function  winmode=Apply window to input  wintype=User defined  sampmode=Continuous  samptime=1  N=64  Rs=50  beta=10  winsamp=Periodic  UserWindow=dpss_return  OptParams=on  UserParams={2}  RowConvenienceOn=on  dataType=double  isSigned=on  wordLen=16  udDataType=sfix(16)  fracBitsMode=Best precision  numFracBits=15  roundingMode=Floor  overflowMode=off  numSidelobes=4  sidelobeLevel=-30
  FFT1 : dspxfrm3/FFT  CompMethod=Table lookup  TableOpt=NEW  TableOptActive=Speed  BitRevOrder=off  InheritFFTLength=on  FFTLength=1024  RowConvenienceOn=on  SkipNorm=off  firstCoeffMode=Specify word length  firstCoeffWordLength=16  firstCoeffFracLength=15  firstCoeffDataTypeStr=fixdt(1,16)  firstCoeffLastDataTypeStr=fixdt(1,16)  outputMin=[]  outputMax=[]  accumDataTypeStr=Inherit: Same as product output  accumLastDataTypeStr=Inherit: Same as product output  roundingMode=Floor  overflowMode=off
  FFT2 : dspxfrm3/FFT  CompMethod=Table lookup  TableOpt=NEW  TableOptActive=Speed  BitRevOrder=off  InheritFFTLength=on  FFTLength=1024  RowConvenienceOn=on  SkipNorm=off  firstCoeffMode=Specify word length  firstCoeffWordLength=16  firstCoeffFracLength=15  firstCoeffDataTypeStr=fixdt(1,16)  firstCoeffLastDataTypeStr=fixdt(1,16)  outputMin=[]  outputMax=[]  accumDataTypeStr=Inherit: Same as product output  accumLastDataTypeStr=Inherit: Same as product output  roundingMode=Floor  overflowMode=off
  Overlap Buffer : Buffer  N=winLen  V=winLen-ana_hopSize  TreatMby1Signals=One channel
  Pad : dspsigops/Pad  padAlong=Columns  dimsToPad=1  valSrc=Specify via dialog  padVal=0  spec=Output size  padNumOutRowsSpecMethod=User-specified  numOutRows=1024  padNumOutColsSpecMethod=User-specified  numOutCols=1  isVarDimsMode=off  padBeginning=0  padEnd=0  outSizeMode=User-specified  outSize=1  padSigAt=Beginning and end  trunc_flag=None  roundingMode=Floor  overflowMode=off  truncOrWrapMode=Truncate  wrap_flag=None
  Pad1 : dspsigops/Pad  padAlong=Columns  dimsToPad=1  valSrc=Specify via dialog  padVal=0  spec=Output size  padNumOutRowsSpecMethod=User-specified  numOutRows=1024  padNumOutColsSpecMethod=User-specified  numOutCols=1  isVarDimsMode=off  padBeginning=0  padEnd=0  outSizeMode=User-specified  outSize=1  padSigAt=Beginning and end  trunc_flag=None  roundingMode=Floor  overflowMode=off  truncOrWrapMode=Truncate  wrap_flag=None
  Out1 : Outport
  Out2 : Outport  Port=2
  Buffer : Outport  Port=3
  wires:
  Overlap Buffer/1 -> Analysis Window/1, Analysis Window1/1, Buffer/1
  FFT1/1 -> Out1/1
  Analysis Window/1 -> Pad/1
  FFT2/1 -> Out2/1
  Analysis Window1/1 -> Pad1/1
  Pad/1 -> FFT1/1
  Pad1/1 -> FFT2/1
  In1/1 -> Overlap Buffer/1

== system test_PCI6251_20130416_3ch/RealSongControl/DSPBlock/SoundOnOffCounter ==
  SoundOn : Inport
  Logical Operator2 : Logic  Operator=NOT  AllPortsSameDT=off  OutDataTypeStr=boolean
  SoundOffCounter : Subsystem
  SoundOnCounter : Subsystem
  SoundONCnt : Outport
  SoundOFFCnt : Outport  Port=2
  wires:
  Logical Operator2/1 -> SoundOffCounter/1(LogicalInput)
  SoundOn/1 -> SoundOnCounter/1(LogicalInput), Logical Operator2/1
  SoundOnCounter/1(count) -> SoundONCnt/1
  SoundOffCounter/1(count) -> SoundOFFCnt/1

== system test_PCI6251_20130416_3ch/RealSongControl/DSPBlock/StimFamilyTriggerButton ==
  Detect Change : simulink/Logic and Bit Operations/Detect Change  SystemSampleTime=-1  vinit=1.0
  TrigVal : Constant  Value=1.0  OutDataTypeStr=int8
  Out1 : Outport
  wires:
  Detect Change/1 -> Out1/1
  TrigVal/1 -> Detect Change/1

== system test_PCI6251_20130416_3ch/RealSongControl/DSPBlock/YIN_FF_estim ==
  In1 : Inport
  DSP Constant1 : Constant  Value=W_index  VectorParams1D=off
  DSP Constant2 : Constant  Value=SampRate  VectorParams1D=off
  DSP Constant3 : Constant  Value=lag_index  VectorParams1D=off
  YIN_FF : Stateflow chart  TreatAsAtomicUnit=on
  FundamentalFrequency : Outport
  wires:
  DSP Constant1/1 -> YIN_FF/3(W_index)
  DSP Constant3/1 -> YIN_FF/4(lag_index)
  In1/1 -> YIN_FF/1(x)
  YIN_FF/1(F0) -> FundamentalFrequency/1
  DSP Constant2/1 -> YIN_FF/2(Fs)

== system test_PCI6251_20130416_3ch/RealSongControl/TriggerCounter/Counter ==
  In1 : Inport
  Enable : EnablePort
  Memory1 : Memory  InheritSampleTime=on
  Sum1 : Sum  Inputs=|++  SaturateOnIntegerOverflow=on
  Out1 : Outport  InitialOutput=0
  wires:
  In1/1 -> Sum1/1
  Sum1/1 -> Out1/1, Memory1/1
  Memory1/1 -> Sum1/2

== system test_PCI6251_20130416_3ch/RealSongControl/DSPBlock/BoutCounter/BoutDurCounter ==
  Input : Inport
  threshold : Inport  Port=2
  CorrectDelayedPulseGenerator ForSyllableOn : Subsystem  mask{maindetection_startcnt=0, width=mingap}
      mask prompts: maindetection_startcnt "Delay (count)"; width "Width of TTL (count)"
  DSP Constant2 : Constant  Value=minsyl  VectorParams1D=off
  PreSoundOnCounter : Subsystem
  Relational Operator : RelationalOperator  Operator=>  OutDataTypeStr=boolean
  Relational Operator1 : RelationalOperator  Operator=>  OutDataTypeStr=boolean
  SoundOnCounter : Subsystem
  SignalOn : Outport
  SignalOnCnt : Outport  Port=2
  wires:
  Relational Operator/1 -> CorrectDelayedPulseGenerator ForSyllableOn/1(trig)
  Input/1 -> Relational Operator/1
  threshold/1 -> Relational Operator/2
  CorrectDelayedPulseGenerator ForSyllableOn/1(TTL) -> PreSoundOnCounter/1(LogicalInput)
  PreSoundOnCounter/1(count) -> Relational Operator1/1
  Relational Operator1/1 -> SignalOn/1, SoundOnCounter/1(LogicalInput)
  DSP Constant2/1 -> Relational Operator1/2
  SoundOnCounter/1(count) -> SignalOnCnt/1

== system test_PCI6251_20130416_3ch/RealSongControl/DSPBlock/BoutCounter/CorrectDelayedPulseGenerator forRecordingEnableSignal ==
  trig : Inport
  DSP Constant2 : Constant  Value=maindetection_startcnt  VectorParams1D=off
  DSP Constant3 : Constant  Value=width  VectorParams1D=off
  Delayed TTL generator : Stateflow chart  TreatAsAtomicUnit=on
  TTL : Outport
  wires:
  DSP Constant2/1 -> Delayed TTL generator/2(delays)
  DSP Constant3/1 -> Delayed TTL generator/3(width)
  trig/1 -> Delayed TTL generator/1(trig)
  Delayed TTL generator/1(out) -> TTL/1

== system test_PCI6251_20130416_3ch/RealSongControl/DSPBlock/FeatureBasedTrigger/MainDetectCounter ==
  LogicalInput : Inport
  Counter : Subsystem  TreatAsAtomicUnit=on
  Data Type Conversion1 : DataTypeConversion  OutDataTypeStr=double  RndMeth=Zero
  count : Outport
  wires:
  Data Type Conversion1/1 -> Counter/1(In1)
  LogicalInput/1 -> Data Type Conversion1/1, Counter/Enable
  Counter/1(Out1) -> count/1

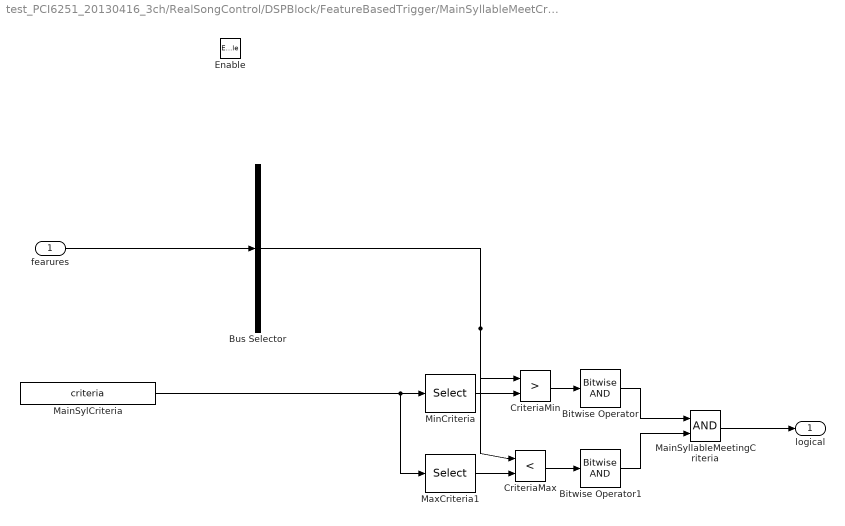
== system test_PCI6251_20130416_3ch/RealSongControl/DSPBlock/FeatureBasedTrigger/MainSyllableMeetCriteria ==
  fearures : Inport
  Enable : EnablePort
  Bitwise Operator : simulink/Logic and Bit Operations/Bitwise Operator  logicop=AND  UseBitMask=off  BitMask=bin2dec('11011001')  BitMaskRealWorld=Stored Integer
  Bitwise Operator1 : simulink/Logic and Bit Operations/Bitwise Operator  logicop=AND  UseBitMask=off  BitMask=bin2dec('11011001')  BitMaskRealWorld=Stored Integer
  Bus Selector : BusSelector  OutputSignals=m_amplitude,signal2.m_Entropy,signal2.m_frequency,signal2.m_FM,signal2.m_Pitch,signal2.m_PitchGoodness,m_PrecisePitch,F0  OutputAsBus=on
  CriteriaMax : RelationalOperator  Operator=<  OutDataTypeStr=boolean
  CriteriaMin : RelationalOperator  Operator=>  OutDataTypeStr=boolean
  MainSylCriteria : Constant  Value=criteria  VectorParams1D=off
  MainSyllableMeetingCriteria : Logic  AllPortsSameDT=off  OutDataTypeStr=boolean
  MaxCriteria1 : Selector  NumberOfDimensions=2  InputPortWidth=3  IndexOptions=Select all,Index vector (dialog)  Indices=[1 3],2  OutputSizes=1,1
  MinCriteria : Selector  NumberOfDimensions=2  InputPortWidth=3  IndexOptions=Select all,Index vector (dialog)  Indices=[1 3],1  OutputSizes=1,1
  logical : Outport  OutputWhenDisabled=reset  InitialOutput=0
  wires:
  fearures/1 -> Bus Selector/1
  MainSylCriteria/1 -> MinCriteria/1, MaxCriteria1/1
  Bus Selector/1 -> CriteriaMin/1, CriteriaMax/1
  MinCriteria/1 -> CriteriaMin/2
  MaxCriteria1/1 -> CriteriaMax/2
  CriteriaMin/1 -> Bitwise Operator/1
  CriteriaMax/1 -> Bitwise Operator1/1
  Bitwise Operator/1 -> MainSyllableMeetingCriteria/1
  Bitwise Operator1/1 -> MainSyllableMeetingCriteria/2
  MainSyllableMeetingCriteria/1 -> logical/1

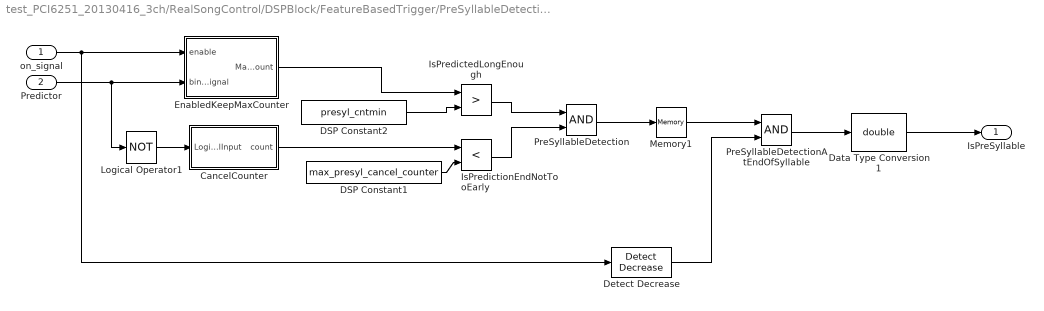
== system test_PCI6251_20130416_3ch/RealSongControl/DSPBlock/FeatureBasedTrigger/PreSyllableDetectionAtEndOfSyllable ==
  on_signal : Inport
  Predictor : Inport  Port=2
  CancelCounter : Subsystem
  DSP Constant1 : Constant  Value=max_presyl_cancel_counter  VectorParams1D=off
  DSP Constant2 : Constant  Value=presyl_cntmin  VectorParams1D=off
  Data Type Conversion1 : DataTypeConversion  OutDataTypeStr=double  RndMeth=Zero
  Detect Decrease : simulink/Logic and Bit Operations/Detect Decrease  SystemSampleTime=-1  vinit=0.0
  EnabledKeepMaxCounter : Subsystem
  IsPredictedLongEnough : RelationalOperator  Operator=>  OutDataTypeStr=boolean
  IsPredictionEndNotTooEarly : RelationalOperator  Operator=<  OutDataTypeStr=boolean
  Logical Operator1 : Logic  Operator=NOT  AllPortsSameDT=off  OutDataTypeStr=boolean
  Memory1 : Memory  InheritSampleTime=on
  PreSyllableDetection : Logic  AllPortsSameDT=off  OutDataTypeStr=boolean
  PreSyllableDetectionAtEndOfSyllable : Logic  AllPortsSameDT=off  OutDataTypeStr=boolean
  IsPreSyllable : Outport
  wires:
  EnabledKeepMaxCounter/1(MaxCount) -> IsPredictedLongEnough/1
  Logical Operator1/1 -> CancelCounter/1(LogicalInput)
  CancelCounter/1(count) -> IsPredictionEndNotTooEarly/1
  DSP Constant2/1 -> IsPredictedLongEnough/2
  IsPredictedLongEnough/1 -> PreSyllableDetection/1
  IsPredictionEndNotTooEarly/1 -> PreSyllableDetection/2
  PreSyllableDetection/1 -> Memory1/1
  on_signal/1 -> EnabledKeepMaxCounter/1(enable), Detect Decrease/1
  Predictor/1 -> EnabledKeepMaxCounter/2(binarysignal), Logical Operator1/1
  DSP Constant1/1 -> IsPredictionEndNotTooEarly/2
  Memory1/1 -> PreSyllableDetectionAtEndOfSyllable/1
  PreSyllableDetectionAtEndOfSyllable/1 -> Data Type Conversion1/1
  Detect Decrease/1 -> PreSyllableDetectionAtEndOfSyllable/2
  Data Type Conversion1/1 -> IsPreSyllable/1

== system test_PCI6251_20130416_3ch/RealSongControl/DSPBlock/FeatureBasedTrigger/ResettableSyllableCounter ==
  sound_on : Inport
  reset : Inport  Port=2
  Detect Increase : simulink/Logic and Bit Operations/Detect Increase  SystemSampleTime=-1  vinit=0.0
  MATLAB Function : Stateflow chart  TreatAsAtomicUnit=on
  "#Syllable since last reset " : Outport
  wires:
  Detect Increase/1 -> MATLAB Function/1(x)
  sound_on/1 -> Detect Increase/1
  MATLAB Function/1(y) -> "#Syllable since last reset "/1
  reset/1 -> MATLAB Function/2(reset)

== system test_PCI6251_20130416_3ch/RealSongControl/DSPBlock/FeatureBasedTrigger/RndCatchMainGateWindow ==
  In1 : Inport
  CorrectDelayedPulseGenerator : Subsystem  mask{maindetection_startcnt=maindetection_startcnt, width=maindetection_endcnt-maindetection_startcnt}
      mask prompts: maindetection_startcnt "Delay (count)"; width "Width of TTL (count)"
  CorrectDelayedPulseGenerator1 : Subsystem  mask{maindetection_startcnt=maindetection_startcnt, width=maindetection_endcnt-maindetection_startcnt}
      mask prompts: maindetection_startcnt "Delay (count)"; width "Width of TTL (count)"
  EnabledCatchSignalBox : Subsystem  TreatAsAtomicUnit=on
  MainTrig_Delay : Constant  Value=maindetection_startcnt  VectorParams1D=off
  MainTrig_Width : Constant  Value=maindetection_endcnt-maindetection_startcnt  VectorParams1D=off
  Hit : Outport
  Catch : Outport  Port=2
  wires:
  EnabledCatchSignalBox/1(Hit) -> CorrectDelayedPulseGenerator/1(trig)
  In1/1 -> EnabledCatchSignalBox/1(In1), EnabledCatchSignalBox/Enable
  CorrectDelayedPulseGenerator/1(TTL) -> Hit/1
  CorrectDelayedPulseGenerator1/1(TTL) -> Catch/1
  EnabledCatchSignalBox/2(Catch) -> CorrectDelayedPulseGenerator1/1(trig)
  MainTrig_Delay/1 -> CorrectDelayedPulseGenerator/2(delay), CorrectDelayedPulseGenerator1/2(delay)
  MainTrig_Width/1 -> CorrectDelayedPulseGenerator/3(width), CorrectDelayedPulseGenerator1/3(width)

== system test_PCI6251_20130416_3ch/RealSongControl/DSPBlock/FeatureBasedTrigger/Spectrum_based_MainSylDetection ==
  m_PowSpec : Inport
  Do_Use_Spectrum_Based_SylDetection : Inport  Port=2
  Logic_spec : Logic  Operator=OR  AllPortsSameDT=off  OutDataTypeStr=boolean
  Logic_spec1 : Logic  Operator=NOT  AllPortsSameDT=off  OutDataTypeStr=boolean
  Product : Product  RndMeth=Zero
  Spectrum_Filter_Constant : Constant  Value=maintarget_spectrum_filter
  Spectrum_Filter_Threshold : Constant  Value=Spectrum_Filter_Threshold
  Spectrum_based_discrimination : RelationalOperator  OutDataTypeStr=boolean
  Sum : Sum  Inputs=+
  Spectrum_Matched : Outport
  SpectCorr : Outport  Port=2
  wires:
  Product/1 -> Sum/1
  Spectrum_Filter_Constant/1 -> Product/2
  Sum/1 -> Spectrum_based_discrimination/1, SpectCorr/1
  Spectrum_Filter_Threshold/1 -> Spectrum_based_discrimination/2
  m_PowSpec/1 -> Product/1
  Spectrum_based_discrimination/1 -> Logic_spec/1
  Logic_spec/1 -> Spectrum_Matched/1
  Do_Use_Spectrum_Based_SylDetection/1 -> Logic_spec1/1
  Logic_spec1/1 -> Logic_spec/2
